simulink model "AircraftModel"  (R2021a)
settings: Solver=VariableStepAuto  StartTime=0.0  StopTime=10  RelTol=1e-3
model workspace: external: MATLAB File C:\Users\SuturinDA\Desktop\course\Model\Parameters.m (data not in the file)
values from neighbouring files (symbols this model uses):
  BatteryVoltage = 44.4    [Parameters.m]
  CQ0 = 0.005230    (= 0.00523)    [Parameters.m]
  CQ1 = 0.004970    (= 0.00497)    [Parameters.m]
  CQ2 = -0.01664    [Parameters.m]
  CT0 = 0.09357    [Parameters.m]
  CT1 = -0.06044    [Parameters.m]
  CT2 = -0.1079    [Parameters.m]
  Dprop = 0.508    [Parameters.m]
  G1 = Jxz*(Jx-Jy+Jz)/G    (= 0.121085757929)    [Parameters.m]
  G2 = (Jz*(Jz-Jy)+Jxz*Jxz)/G    (= 0.77491540164)    [Parameters.m]
  G5 = (Jz-Jx)/Jy    (= 0.823788546256)    [Parameters.m]
  G6 = Jxz/Jy    (= 0.105726872247)    [Parameters.m]
  G7 = ((Jx-Jy)*Jx + Jxz*Jxz) / G    (= -0.168544462222)    [Parameters.m]
  i0 = 1.5    [Parameters.m]
  KQ = 0.0659    [Parameters.m]
  KV = 0.0659    [Parameters.m]
  MotorPosition = [-0.15; 0; 0]    [Parameters.m]
  Rmotor = 0.042    [Parameters.m]
  WGS84_a = 6378137.0    (= 6378137)    [Parameters.m]
  WGS84_e1 = sqrt((WGS84_a*WGS84_a - WGS84_b*WGS84_b) / (WGS84_a*WGS84_a))    [Parameters.m]
  WGS84_FlatteningFactor = 298.257223563    [Parameters.m]
  WGS84_GravityConstant = 1.931852652458e-3    (= 0.00193185265246)    [Parameters.m]
  WGS84_GravityEquator = 9.7803253359    [Parameters.m]
  WGS84_m = (WGS84_w * WGS84_a)^2 * WGS84_b / WGS84_GM    (= 0.00344978650684)    [Parameters.m]
undefined symbols (not defined in the file or in its folder): param
libraries: aerosimlib x4, vrlib x1, sharedutil x1, matrix_library x1
settings Model: Creator=SuturinDA  LastModifiedBy=PC

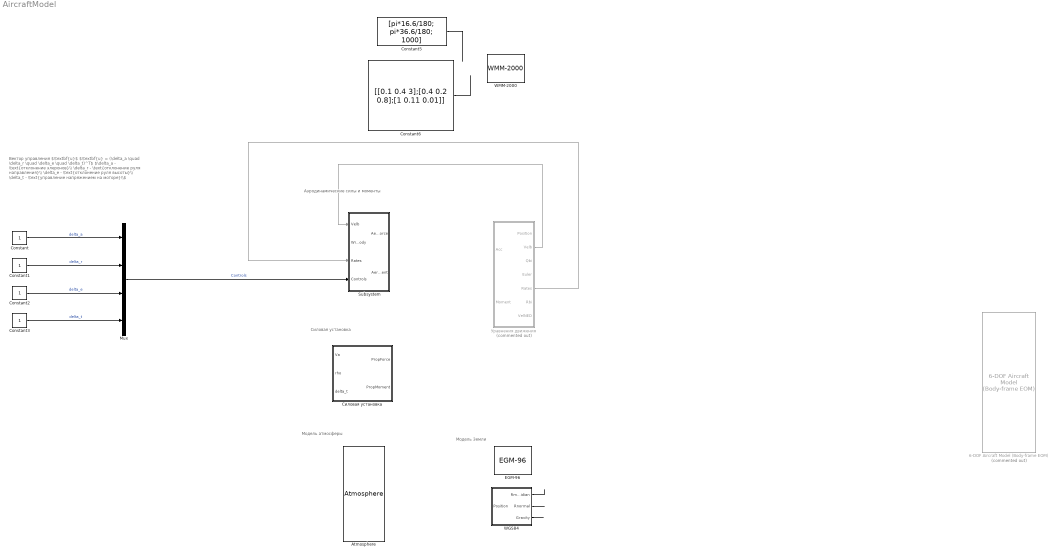
== system AircraftModel ==
  note: Вектор управления $\textbf{u}$
      | $\textbf{u} = (\delta_a \quad \delta_r \quad \delta_e \quad \delta_t)^T$
      | $\delta_a - \text{отклонение элеронов}\\ \delta_r - \text{отклонение руля направления}\\ \delta_e - \text{отклонение руля высоты}\\ \delta_t - \text{управление напряжением на моторе}\\$
  note: Модель Земли
  note: Модель атмосферы
  note: Силовая установка
  note: Аэродинамические силы и моменты
  6-DOF Aircraft Model (Body-frame EOM) : aerosimlib/Complete Aircraft/6-DOF Aircraft Model (Body-frame EOM)  Commented=on  aircraftcfg='unknown.mat'  VelocitiesIni=[0 0 0]'  RatesIni=[0 0 0]'  QuaternionsIni=[1 0 0 0]'  PositionIni=[0*pi/180 0*pi/180 0]'  FuelIni=0  OmegaIni=0*pi/30  GndAlt=0  wmmfile='c:\Program Files\AeroSim\wmm.cof'  dmy=[08 01 2004]  tsamp=0.005
      settings: SourceProductName=AeroSim Blockset
  Atmosphere : aerosimlib/Complete Aircraft/6-DOF Aircraft Model (Body-frame EOM)/Atmosphere  SystemSampleTime=-1  VariantActivationTime=update diagram  Latency=0  AutoFrameSizeCalculation=off
      settings: SourceProductName=AeroSim Blockset
  Constant{,1..3} (4 alike) : Constant
  Constant5 : Constant  Value=[pi*16.6/180; pi*36.6/180; 1000]
  Constant6 : Constant  Value=[[0.1 0.4 3];[0.4 0.2 0.8];[1 0.11 0.01]]
  EGM-96 : aerosimlib/Earth/EGM-96
      settings: SourceProductName=AeroSim Blockset
  Mux : Mux
  Subsystem : Subsystem
  WGS84 : Subsystem
  WMM-2000 : aerosimlib/Earth/WMM-2000  wmmfile='c:\Program Files (x86)\AeroSim\wmm.cof'  simdate=[1 12 2025]
      link override S-Function: FunctionName=sfunwmm
      settings: SourceProductName=AeroSim Blockset
  Силовая установка : Subsystem
  Уравнения движения : Subsystem  Commented=on
  wires:
  Constant/1 -> Mux/1  "delta_a"
  Constant1/1 -> Mux/2  "delta_r"
  Constant2/1 -> Mux/3  "delta_e"
  Constant3/1 -> Mux/4  "delta_t"
  Mux/1 -> Subsystem/4(Controls)  "Controls"
  Уравнения движения/5(Rates) -> Subsystem/3(Rates)
  Уравнения движения/2(Velb) -> Subsystem/1(Velb)
  WGS84/2(Rnormal) -> ?
  WGS84/1(Rmeridian) -> ?
  WGS84/3(Gravity) -> ?
  Constant5/1 -> ?
  Constant6/1 -> ?

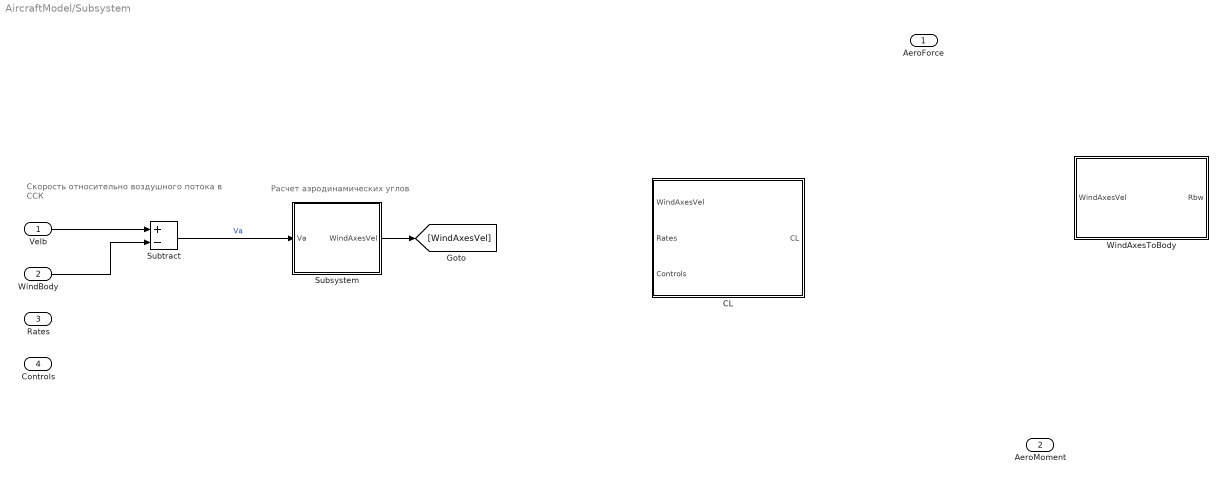
== system AircraftModel/Subsystem ==
  note: Расчет аэродинамических углов
  note: Скорость относительно воздушного потока
      | в ССК
  Velb : Inport
  WindBody : Inport  Port=2
  Rates : Inport  Port=3
  Controls : Inport  Port=4
  CL : Subsystem
  Subsystem : Subsystem
  Subtract : Sum  Inputs=+-
  WindAxesToBody : MATLAB Function  TreatAsAtomicUnit=on
  AeroForce : Outport
  AeroMoment : Outport  Port=2
  wires:
  Velb/1 -> Subtract/1
  WindBody/1 -> Subtract/2
  Subtract/1 -> Subsystem/1(Va)  "Va"
  Subsystem/1(WindAxesVel) -> [WindAxesVel]

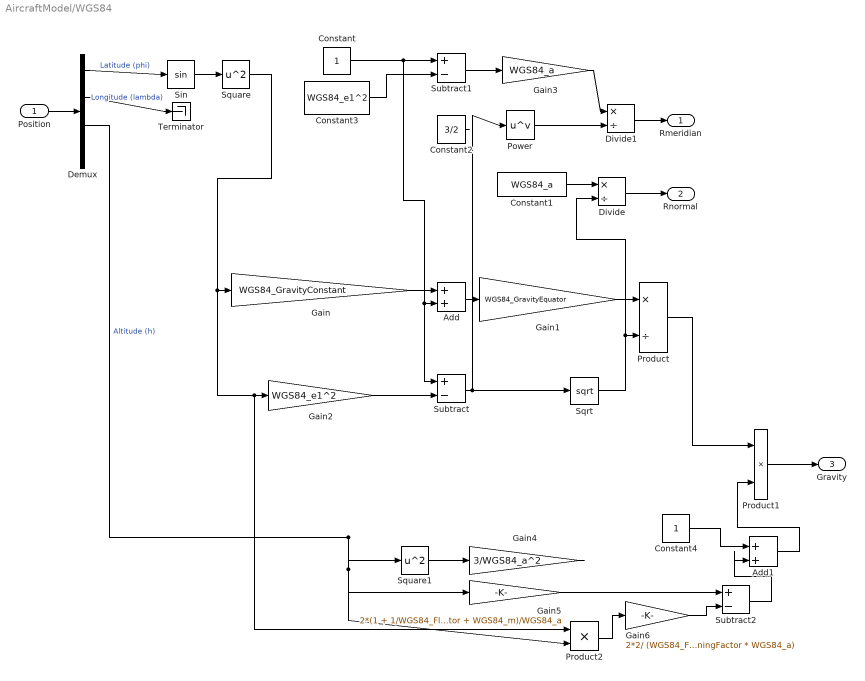
== system AircraftModel/WGS84 ==
  Position : Inport
  Add : Sum
  Add1 : Sum  Inputs=+-+
  Constant : Constant
  Constant1 : Constant  Value=WGS84_a
  Constant2 : Constant  Value=3/2
  Constant3 : Constant  Value=WGS84_e1^2
  Constant4 : Constant
  Demux : Demux  Outputs=3
  Divide : Product  Inputs=*/
  Divide1 : Product  Inputs=*/
  Gain : Gain  Gain=WGS84_GravityConstant
  Gain1 : Gain  Gain=WGS84_GravityEquator
  Gain2 : Gain  Gain=WGS84_e1^2
  Gain3 : Gain  Gain=WGS84_a
  Gain4 : Gain  Gain=3/WGS84_a^2
  Gain5 : Gain  Gain=2*(1 + 1/WGS84_FlatteningFactor + WGS84_m)/WGS84_a
  Gain6 : Gain  Gain=2*2/ (WGS84_FlatteningFactor * WGS84_a)
  Power : Math  Operator=pow  SignedPower=on  SaturateOnIntegerOverflow=on
  Product : Product  Inputs=*/
  Product1 : Product
  Product2 : Product
  Sin : Trigonometry
  Sqrt : Sqrt  SaturateOnIntegerOverflow=on
  Square : Math  Operator=square  SaturateOnIntegerOverflow=on
  Square1 : Math  Operator=square  SaturateOnIntegerOverflow=on
  Subtract : Sum  Inputs=+-
  Subtract1 : Sum  Inputs=+-
  Subtract2 : Sum  Inputs=+-
  Terminator : Terminator
  Rmeridian : Outport
  Rnormal : Outport  Port=2
  Gravity : Outport  Port=3
  wires:
  Position/1 -> Demux/1
  Demux/1 -> Sin/1  "Latitude (phi)"
  Demux/2 -> Terminator/1  "Longitude (lambda)"
  Demux/3 -> Square1/1, Gain5/1, Product2/2  "Altitude (h)"
  Sin/1 -> Square/1
  Product/1 -> Product1/1
  Constant/1 -> Subtract/1, Add/2, Subtract1/1
  Add/1 -> Gain1/1
  Gain/1 -> Add/1
  Square/1 -> Product2/1, Gain2/1, Gain/1
  Gain1/1 -> Product/1
  Sqrt/1 -> Divide/2, Product/2
  Subtract/1 -> Sqrt/1, Power/1
  Gain2/1 -> Subtract/2
  Divide/1 -> Rnormal/1
  Constant1/1 -> Divide/1
  Divide1/1 -> Rmeridian/1
  Power/1 -> Divide1/2
  Constant2/1 -> ?
  Subtract1/1 -> Gain3/1
  Gain3/1 -> Divide1/1
  Constant3/1 -> Subtract1/2
  Product1/1 -> Gravity/1
  Square1/1 -> Gain4/1
  Gain5/1 -> Subtract2/1
  Product2/1 -> Gain6/1
  Gain6/1 -> Subtract2/2
  Constant4/1 -> Add1/1
  Subtract2/1 -> Add1/2
  Gain4/1 -> ?
  Add1/1 -> Product1/2

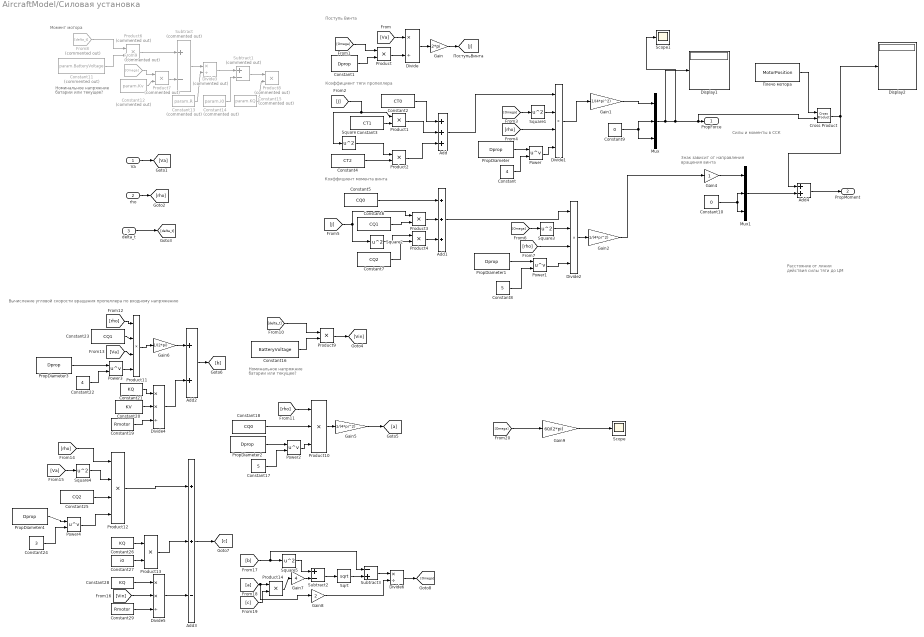
== system AircraftModel/Силовая установка ==
  note: Вычисление угловой скорости вращения пропеллера по входному напряжению
  note: Момент мотора
  note: Номинальное напряжние
      | батарии или текущее?
  note: Знак зависит от направления
      | вращения винта
  note: Силы и моменты в ССК
  note: Расстояние от линии
      | действия силы тяги до ЦМ
  note: Коэффициент момента винта
  note: Коэффициент тяги пропеллера
  note: Поступь Винта
  note: Номинальное напряжние
      | батарии или текущее?
  Va : Inport
  rho : Inport  Port=2
  delta_t : Inport  Port=3
  Add : Sum  Inputs=+++
  Add1 : Sum  Inputs=+++
  Add2 : Sum
  Add3 : Sum  Inputs=++-
  Add4 : Sum
  Constant : Constant  Value=4
  Constant1 : Constant  Value=Dprop
  Constant10 : Constant  Value=0
  Constant11 : Constant  Commented=on  Value=param.BatteryVoltage
  Constant12 : Constant  Commented=on  Value=param.Kv
  Constant13 : Constant  Commented=on  Value=param.R
  Constant14 : Constant  Commented=on  Value=param.i0
  Constant15 : Constant  Commented=on  Value=param.KQ
  Constant16 : Constant  Value=BatteryVoltage
  Constant17 : Constant  Value=5
  Constant18 : Constant  Value=CQ0
  Constant19 : Constant  Value=Rmotor
  Constant2 : Constant  Value=CT0
  Constant20 : Constant  Value=KV
  Constant21 : Constant  Value=KQ
  Constant22 : Constant  Value=4
  Constant23 : Constant  Value=CQ1
  Constant24 : Constant  Value=3
  Constant25 : Constant  Value=CQ2
  Constant26 : Constant  Value=KQ
  Constant27 : Constant  Value=i0
  Constant28 : Constant  Value=KQ
  Constant29 : Constant  Value=Rmotor
  Constant3 : Constant  Value=CT1
  Constant4 : Constant  Value=CT2
  Constant5 : Constant  Value=CQ0
  Constant6 : Constant  Value=CQ1
  Constant7 : Constant  Value=CQ2
  Constant8 : Constant  Value=5
  Constant9 : Constant  Value=0
  Cross Product : vrlib/Utilities/Cross Product
  Display1 : Display
  Display2 : Display
  Divide : Product  Inputs=*/
  Divide1 : Product  Inputs=****
  Divide2 : Product  Inputs=****
  Divide3 : Product  Commented=on  Inputs=*/
  Divide4 : Product  Inputs=**/
  Divide5 : Product  Inputs=**/
  Divide6 : Product  Inputs=*/
  From8 : From  Commented=on  GotoTag=delta_t
  From9 : From  Commented=on  GotoTag=Omega
  Gain : Gain  Gain=2*pi
  Gain1 : Gain  Gain=1/(4*pi^2)
  Gain2 : Gain  Gain=1/(4*pi^2)
  Gain4 : Gain
  Gain5 : Gain  Gain=1/(4*pi^2)
  Gain6 : Gain  Gain=1/(2*pi)
  Gain7 : Gain  Gain=4
  Gain8 : Gain  Gain=2
  Gain9 : Gain  Gain=60/(2*pi)
  Mux : Mux  Inputs=3
  Mux1 : Mux  Inputs=3
  Power{,1..4} (5 alike) : Math  Operator=pow  SaturateOnIntegerOverflow=on
  Product{,1..4,9,13..14} (8 alike) : Product
  Product10 : Product  Inputs=3
  Product11 : Product  Inputs=4
  Product12 : Product  Inputs=4
  Product6 : Product  Commented=on
  Product7 : Product  Commented=on
  Product8 : Product  Commented=on
  PropDiameter{,1..4} (5 alike) : Constant  Value=Dprop
  Scope : Scope
  Scope1 : Scope
  Sqrt : Sqrt  SaturateOnIntegerOverflow=on
  Square{,1..5} (6 alike) : Math  Operator=square  SaturateOnIntegerOverflow=on
  Subtract : Sum  Commented=on  Inputs=+-
  Subtract1 : Sum  Commented=on  Inputs=+-
  Subtract2 : Sum  Inputs=+-
  Subtract3 : Sum  Inputs=-+
  Плечо мотора : Constant  Value=MotorPosition
  PropForce : Outport
  PropMoment : Outport  Port=2
  wires:
  Constant/1 -> Power/2
  Va/1 -> [Va]
  Divide/1 -> Gain/1
  Gain/1 -> [J]
  [Va] -> Divide/1
  Product/1 -> Divide/2
  [Omega] -> Product/1
  Constant1/1 -> Product/2
  rho/1 -> [rho]
  Product1/1 -> Add/2
  Product2/1 -> Add/3
  Constant2/1 -> Add/1
  Constant3/1 -> Product1/2
  Constant4/1 -> Product2/2
  [J] -> Product1/1, Square/1
  Square/1 -> Product2/1
  Divide1/1 -> Gain1/1
  Add/1 -> Divide1/1
  [Omega] -> Square1/1
  Square1/1 -> Divide1/2
  Constant5/1 -> Add1/1
  Product3/1 -> Add1/2
  [J] -> Product3/1, Square2/1
  Constant6/1 -> Product3/2
  Constant7/1 -> Product4/2
  Square2/1 -> Product4/1
  Add1/1 -> Divide2/1
  [Omega] -> Square3/1
  Square3/1 -> Divide2/2
  Divide2/1 -> Gain2/1
  Constant8/1 -> Power1/2
  PropDiameter1/1 -> Power1/1
  Mux/1 -> Scope1/1, Cross Product/2, PropForce/1, Display1/1
  Gain1/1 -> Mux/1
  Constant9/1 -> Mux/2, Mux/3
  Gain2/1 -> Gain4/1
  Mux1/1 -> Add4/2
  Плечо мотора/1 -> Cross Product/1
  Constant10/1 -> Mux1/3, Mux1/2
  Gain4/1 -> Mux1/1
  delta_t/1 -> [delta_t]
  Constant11/1 -> Product6/2
  From8/1 -> Product6/1
  Product6/1 -> Subtract/1
  Product7/1 -> Subtract/2
  Constant12/1 -> Product7/2
  From9/1 -> Product7/1
  Subtract/1 -> Divide3/1
  Constant13/1 -> Divide3/2
  Divide3/1 -> Subtract1/1
  Constant14/1 -> Subtract1/2
  Subtract1/1 -> Product8/1
  Constant15/1 -> Product8/2
  Constant16/1 -> Product9/2
  [delta_t] -> Product9/1
  Product9/1 -> [Vin]
  [rho] -> Product10/1
  Constant17/1 -> Power2/2
  Constant18/1 -> Product10/2
  Product10/1 -> Gain5/1
  Gain5/1 -> [a]
  Divide4/1 -> Add2/2
  Constant19/1 -> Divide4/3
  Constant20/1 -> Divide4/2
  Constant21/1 -> Divide4/1
  Product11/1 -> Gain6/1
  Gain6/1 -> Add2/1
  [rho] -> Product11/1
  Constant22/1 -> Power3/2
  PropDiameter3/1 -> Power3/1
  Constant23/1 -> Product11/2
  Add2/1 -> [b]
  Product12/1 -> Add3/1
  [rho] -> Product12/1
  Constant24/1 -> Power4/2
  PropDiameter4/1 -> Power4/1
  [Va] -> Square4/1
  Square4/1 -> Product12/2
  Product13/1 -> Add3/2
  Constant26/1 -> Product13/1
  Constant27/1 -> Product13/2
  Constant28/1 -> Divide5/1
  [Vin] -> Divide5/2
  Add3/1 -> [c]
  [b] -> Subtract3/1, Square5/1
  Square5/1 -> Subtract2/1
  [a] -> Product14/1, Gain8/1
  [c] -> Product14/2
  Product14/1 -> Gain7/1
  Subtract2/1 -> Sqrt/1
  Sqrt/1 -> Subtract3/2
  Gain7/1 -> Subtract2/2
  Subtract3/1 -> Divide6/1
  Gain8/1 -> Divide6/2
  Divide6/1 -> [Omega]
  [Omega] -> Gain9/1
  Gain9/1 -> Scope/1
  Add4/1 -> PropMoment/1
  Product4/1 -> Add1/3
  PropDiameter2/1 -> Power2/1
  Power2/1 -> Product10/3
  [Va] -> Product11/3
  Power3/1 -> Product11/4
  Constant25/1 -> Product12/3
  Power4/1 -> Product12/4
  Constant29/1 -> Divide5/3
  Divide5/1 -> Add3/3
  [rho] -> Divide2/3
  Power1/1 -> Divide2/4
  PropDiameter/1 -> Power/1
  Power/1 -> Divide1/4
  [rho] -> Divide1/3
  Cross Product/1 -> Display2/1, Add4/1

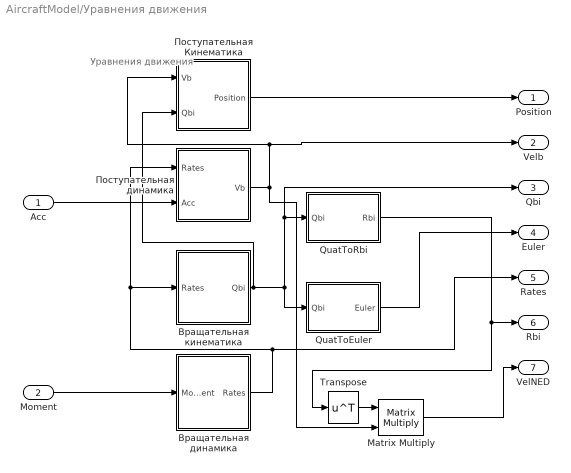
== system AircraftModel/Уравнения движения ==
  note: Уравнения движения
  Acc : Inport
  Moment : Inport  Port=2
  Matrix Multiply : Product  Multiplication=Matrix(*)
  QuatToEuler : MATLAB Function  TreatAsAtomicUnit=on
  QuatToRbi : MATLAB Function  TreatAsAtomicUnit=on
  Transpose : Math  Operator=transpose  SaturateOnIntegerOverflow=on
  Вращательная динамика : Subsystem
  Вращательная кинематика : Subsystem
  Поступательная Кинематика : Subsystem
  Поступательная динамика : Subsystem
  Position : Outport
  Velb : Outport  Port=2
  Qbi : Outport  Port=3
  Euler : Outport  Port=4
  Rates : Outport  Port=5
  Rbi : Outport  Port=6
  VelNED : Outport  Port=7
  wires:
  Вращательная кинематика/1(Qbi) -> Поступательная Кинематика/2(Qbi), QuatToEuler/1(Qbi), QuatToRbi/1(Qbi), Qbi/1
  Вращательная динамика/1(Rates) -> Rates/1, Вращательная кинематика/1(Rates), Поступательная динамика/1(Rates)
  Acc/1 -> Поступательная динамика/2(Acc)
  QuatToRbi/1(Rbi) -> Transpose/1, Rbi/1
  Поступательная динамика/1(Vb) -> Matrix Multiply/2, Velb/1, Поступательная Кинематика/1(Vb)
  QuatToEuler/1(Euler) -> Euler/1
  Moment/1 -> Вращательная динамика/1(Moment)
  Поступательная Кинематика/1(Position) -> Position/1
  Transpose/1 -> Matrix Multiply/1
  Matrix Multiply/1 -> VelNED/1

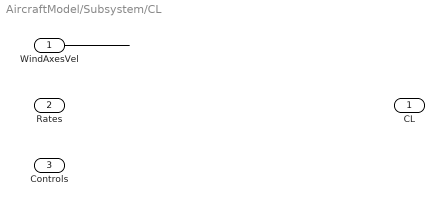
== system AircraftModel/Subsystem/CL ==
  WindAxesVel : Inport
  Rates : Inport  Port=2
  Controls : Inport  Port=3
  CL : Outport
  wires:
  WindAxesVel/1 -> ?

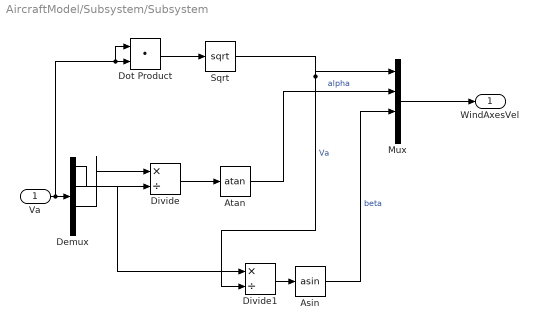
== system AircraftModel/Subsystem/Subsystem ==
  Va : Inport
  Asin : Trigonometry  Operator=asin
  Atan : Trigonometry  Operator=atan
  Demux : Demux  Outputs=3
  Divide : Product  Inputs=*/
  Divide1 : Product  Inputs=*/
  Dot Product : DotProduct  InputSameDT=on  OutDataTypeStr=Inherit: Inherit via internal rule
  Mux : Mux  Inputs=3
  Sqrt : Sqrt  SaturateOnIntegerOverflow=on
  WindAxesVel : Outport
  wires:
  Divide/1 -> Atan/1
  Demux/2 -> Divide1/1
  Atan/1 -> Mux/2  "alpha"
  Va/1 -> Dot Product/1, Dot Product/2, Demux/1
  Mux/1 -> WindAxesVel/1
  Dot Product/1 -> Sqrt/1
  Sqrt/1 -> Divide1/2, Mux/1  "Va"
  Divide1/1 -> Asin/1
  Asin/1 -> Mux/3  "beta"
  Demux/3 -> Divide/1
  Demux/1 -> Divide/2

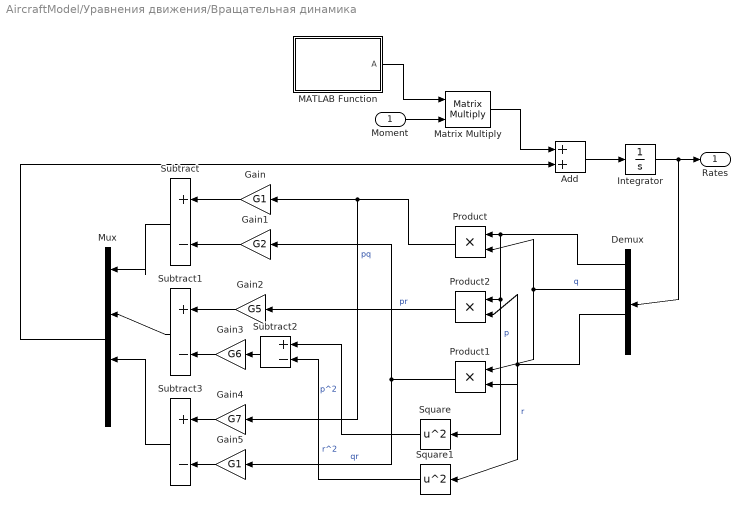
== system AircraftModel/Уравнения движения/Вращательная динамика ==
  Moment : Inport
  Add : Sum
  Demux : Demux  Outputs=3
  Gain : Gain  Gain=G1
  Gain1 : Gain  Gain=G2
  Gain2 : Gain  Gain=G5
  Gain3 : Gain  Gain=G6
  Gain4 : Gain  Gain=G7
  Gain5 : Gain  Gain=G1
  Integrator : Integrator
  MATLAB Function : MATLAB Function  TreatAsAtomicUnit=on
  Matrix Multiply : Product  Multiplication=Matrix(*)
  Mux : Mux  Inputs=3
  Product : Product
  Product1 : Product
  Product2 : Product
  Square : Math  Operator=square  SaturateOnIntegerOverflow=on
  Square1 : Math  Operator=square  SaturateOnIntegerOverflow=on
  Subtract{,1..3} (4 alike) : Sum  Inputs=+-
  Rates : Outport
  wires:
  MATLAB Function/1(A) -> Matrix Multiply/1
  Moment/1 -> Matrix Multiply/2
  Matrix Multiply/1 -> Add/1
  Add/1 -> Integrator/1
  Integrator/1 -> Demux/1, Rates/1
  Demux/1 -> Product2/1, Square/1, Product/1  "p"
  Demux/2 -> Product1/1, Product/2  "q"
  Demux/3 -> Product1/2, Product2/2, Square1/1  "r"
  Product/1 -> Gain/1, Gain4/1  "pq"
  Product1/1 -> Gain5/1, Gain1/1  "qr"
  Product2/1 -> Gain2/1  "pr"
  Square/1 -> Subtract2/1  "p^2"
  Square1/1 -> Subtract2/2  "r^2"
  Gain/1 -> Subtract/1
  Gain1/1 -> Subtract/2
  Gain2/1 -> Subtract1/1
  Gain3/1 -> Subtract1/2
  Subtract2/1 -> Gain3/1
  Gain4/1 -> Subtract3/1
  Gain5/1 -> Subtract3/2
  Subtract/1 -> Mux/1
  Subtract1/1 -> Mux/2
  Subtract3/1 -> Mux/3
  Mux/1 -> Add/2

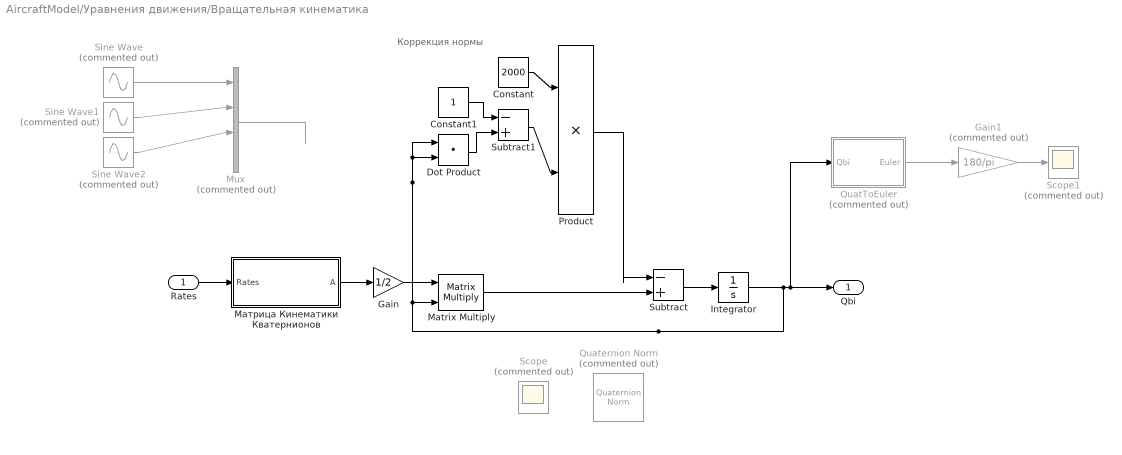
== system AircraftModel/Уравнения движения/Вращательная кинематика ==
  note: Коррекция нормы
  Rates : Inport
  Constant : Constant  Value=2000
  Constant1 : Constant
  Dot Product : DotProduct  InputSameDT=on  OutDataTypeStr=Inherit: Inherit via internal rule
  Gain : Gain  Gain=1/2
  Gain1 : Gain  Commented=on  Gain=180/pi
  Integrator : Integrator  InitialCondition=[1;0;0;0]
  Matrix Multiply : Product  Multiplication=Matrix(*)
  Mux : Mux  Commented=on  Inputs=3
  Product : Product  Inputs=3
  QuatToEuler : MATLAB Function  Commented=on  TreatAsAtomicUnit=on
  Quaternion Norm : sharedutil/Quaternion Norm  Commented=on  aMode=aMode
      settings: SourceProductBaseCode=AE,PW,DR,MT,UV,VE
  Scope : Scope  Commented=on
  Scope1 : Scope  Commented=on
  Sine Wave : Sin  Commented=on  Amplitude=0.01  Frequency=2  SampleTime=0
  Sine Wave1 : Sin  Commented=on  Amplitude=0.02  SampleTime=0
  Sine Wave2 : Sin  Commented=on  Amplitude=0.03  Frequency=5  SampleTime=0
  Subtract : Sum  Inputs=-+
  Subtract1 : Sum  Inputs=-+
  Матрица Кинематики Кватернионов : MATLAB Function  TreatAsAtomicUnit=on
  Qbi : Outport
  wires:
  Rates/1 -> Матрица Кинематики Кватернионов/1(Rates)
  Матрица Кинематики Кватернионов/1(A) -> Gain/1
  Gain/1 -> Matrix Multiply/1
  Integrator/1 -> Dot Product/2, Dot Product/1, Matrix Multiply/2, QuatToEuler/1(Qbi), Qbi/1
  Matrix Multiply/1 -> Subtract/2
  Subtract/1 -> Integrator/1
  Constant/1 -> Product/1
  Product/1 -> Subtract/1
  Constant1/1 -> Subtract1/1
  Dot Product/1 -> Subtract1/2
  Subtract1/1 -> Product/2
  ? -> Scope/1
  Mux/1 -> ?
  Sine Wave/1 -> Mux/1
  Sine Wave1/1 -> Mux/2
  Sine Wave2/1 -> Mux/3
  QuatToEuler/1(Euler) -> Gain1/1
  Gain1/1 -> Scope1/1

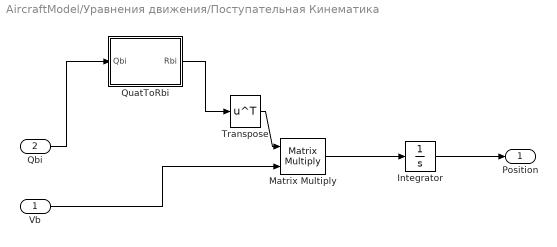
== system AircraftModel/Уравнения движения/Поступательная Кинематика ==
  Vb : Inport
  Qbi : Inport  Port=2
  Integrator : Integrator
  Matrix Multiply : Product  Multiplication=Matrix(*)
  QuatToRbi : MATLAB Function  TreatAsAtomicUnit=on
  Transpose : Math  Operator=transpose  SaturateOnIntegerOverflow=on
  Position : Outport
  wires:
  Vb/1 -> Matrix Multiply/2
  Qbi/1 -> QuatToRbi/1(Qbi)
  QuatToRbi/1(Rbi) -> Transpose/1
  Transpose/1 -> Matrix Multiply/1
  Matrix Multiply/1 -> Integrator/1
  Integrator/1 -> Position/1

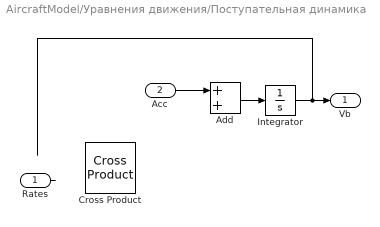
== system AircraftModel/Уравнения движения/Поступательная динамика ==
  Rates : Inport
  Acc : Inport  Port=2
  Add : Sum
  Cross Product : matrix_library/Cross Product
  Integrator : Integrator
  Vb : Outport
  wires:
  Rates/1 -> ?
  Integrator/1 -> Vb/1
  Add/1 -> Integrator/1
  Acc/1 -> Add/1
  ? -> Add/2

== matlab function AircraftModel/Уравнения движения/Вращательная кинематика/Матрица Кинематики Кватернионов ==
  data: Rates input; A output
function A = QuatKinMatrix(Rates)

p = Rates(1);
q = Rates(2);
r = Rates(3);

A = [[0 -p -q -r];
    [p 0 r -q];
    [q -r 0 p];
    [r q -p 0]];
end

== matlab function AircraftModel/Уравнения движения/QuatToEuler ==
  data: Qbi input; Euler output
function Euler = QuatToEuler(Qbi)

q0 = Qbi(1);
q1 = Qbi(2);
q2 = Qbi(3);
q3 = Qbi(4);

phi = atan2(2*(q0*q1+q2*q3), (q0*q0+q3*q3-q1*q1-q2*q2));
theta = asin(2*(q0*q2-q1*q3));
psi = atan2(2*(q0*q3+q1*q2), (q0*q0+q1*q1-q2*q2-q3*q3));

phi = mod(phi + pi, 2*pi) - pi;
theta = mod(theta + pi, 2*pi) - pi;
psi = mod(psi + pi, 2*pi) - pi;

Euler = [phi; theta; psi];

end

== matlab function AircraftModel/Уравнения движения/Поступательная Кинематика/QuatToRbi ==
  data: Qbi input; Rbi output
function Rbi = fcn(Qbi)

q0 = Qbi(1);
q1 = Qbi(2);
q2 = Qbi(3);
q3 = Qbi(4);

Rbi = [[(1-2*q2*q2-2*q3*q3) 2*(q1*q2+q3*q0) 2*(q1*q3-q0*q2)];
    [2*(q1*q2-q3*q0) (q0*q0+q2*q2-q1*q1-q3*q3) 2*(q2*q3+q1*q0)];
    [2*(q1*q3+q0*q2) 2*(q2*q3-q1*q0) (q0*q0+q3*q3-q1*q1-q2*q2)]];
end

== matlab function AircraftModel/Уравнения движения/Вращательная кинематика/QuatToEuler ==
  data: Qbi input; Euler output
function Euler = fcn(Qbi)

q0 = Qbi(1);
q1 = Qbi(2);
q2 = Qbi(3);
q3 = Qbi(4);

phi = atan2(2*(q0*q1+q2*q3), (q0*q0+q3*q3-q1*q1-q2*q2));
theta = asin(2*(q0*q2-q1*q3));
psi = atan2(2*(q0*q3+q1*q2), (q0*q0+q1*q1-q2*q2-q3*q3));

phi = mod(phi + pi, 2*pi) - pi;
theta = mod(theta + pi, 2*pi) - pi;
psi = mod(psi + pi, 2*pi) - pi;

Euler = [phi; theta; psi];

end

== matlab function AircraftModel/Уравнения движения/QuatToRbi ==
  data: Qbi input; Rbi output
function Rbi = QuatToRbi(Qbi)

q0 = Qbi(1);
q1 = Qbi(2);
q2 = Qbi(3);
q3 = Qbi(4);

Rbi = [[(1-2*q2*q2-2*q3*q3) 2*(q1*q2+q3*q0) 2*(q1*q3-q0*q2)];
    [2*(q1*q2-q3*q0) (q0*q0+q2*q2-q1*q1-q3*q3) 2*(q2*q3+q1*q0)];
    [2*(q1*q3+q0*q2) 2*(q2*q3-q1*q0) (q0*q0+q3*q3-q1*q1-q2*q2)]];

== matlab function AircraftModel/Subsystem/WindAxesToBody ==
  data: WindAxesVel input; Rbw output
function Rbw = fcn(WindAxesVel)

Va = WindAxesVel(1);
a = WindAxesVel(2);
b = WindAxesVel(3);

Rbs = [[cos(a) 0 -sin(a)];
    [0 1 0];
    [sin(a) 0 cos(a)]];

Rws = [[cos(b) sin(b) 0];
    [-sin(b) cos(b) 0];
    [0 0 1]];

Rbw = Rbs * Rws';
end

== matlab function AircraftModel/Уравнения движения/Вращательная динамика/MATLAB Function ==
  data: A output
function A = RotDynMatrix()

A = [[G3 0 G4];
    [0 1/Jy 0];
    [G4 0 G8]];
end
